simulink model "Aerodynamics4"  (R2017b)
settings: Solver=ode4  StartTime=0  StopTime=10.0  FixedStep=Ts  RelTol=1e-3
undefined symbols (not defined in the file or in its folder): Actuators, AeroDerivatives, Configuration, magnitude
libraries: aerolibatmos2 x1
settings Model: Creator=zht  LastModifiedBy=zht
settings DataIOCC: SaveFormat=StructureWithTime
settings OptimizationCC: BlockReduction=off  OptimizeBlockIOStorage=off  BufferReuse=off  GlobalBufferReuse=off  ExpressionFolding=off  LocalBlockOutputs=off
settings DebuggingCC: AlgebraicLoopMsg=none  UnconnectedInputMsg=none  UnconnectedOutputMsg=none  UnconnectedLineMsg=none

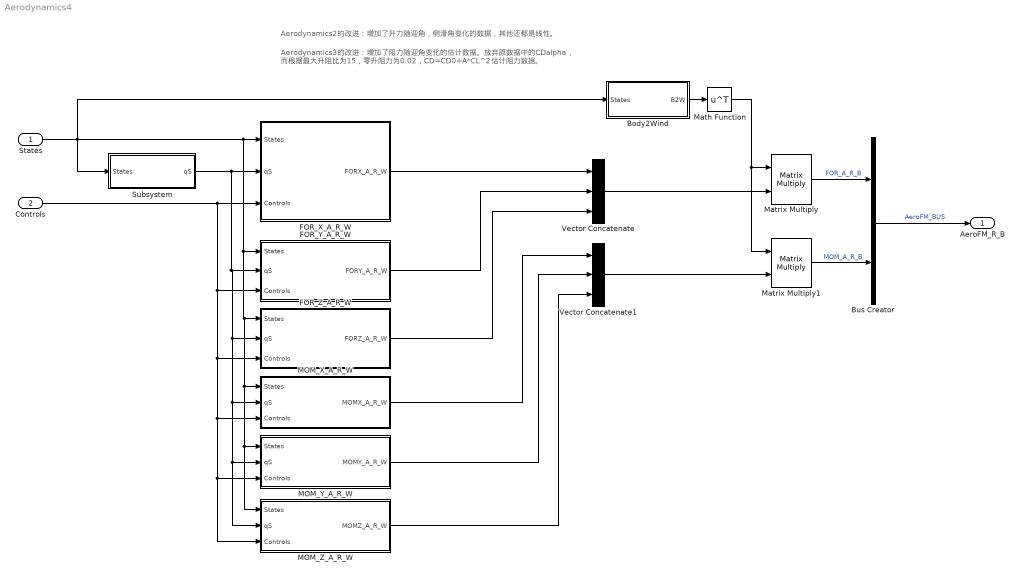
== system Aerodynamics4 ==
  note: Aerodynamics2的改进：增加了升力随迎角，侧滑角变化的数据，其他还都是线性。
  note: Aerodynamics3的改进：增加了阻力随迎角变化的估计数据。放弃原数据中的CDalpha，
      | 而根据最大升阻比为15，零升阻力为0.02，CD=CD0+A*CL^2估计阻力数据。
  States : Inport  OutDataTypeStr=Bus: States_BUS
  Controls : Inport  Port=2  OutDataTypeStr=Bus: Controls_CMD_BUS
  Body2Wind : Subsystem
  Bus Creator : BusCreator  Inputs=2  OutDataTypeStr=Bus: AeroFM_BUS
  FOR_X_A_R_W : Subsystem
  FOR_Y_A_R_W : Subsystem
  FOR_Z_A_R_W : Subsystem
  MOM_X_A_R_W : Subsystem
  MOM_Y_A_R_W : Subsystem
  MOM_Z_A_R_W : Subsystem
  Math Function : Math  Operator=transpose  SaturateOnIntegerOverflow=on
  Matrix Multiply : Product  Multiplication=Matrix(*)
  Matrix Multiply1 : Product  Multiplication=Matrix(*)
  Subsystem : Subsystem
  Vector Concatenate : Concatenate  NumInputs=3  Mode=Multidimensional array
  Vector Concatenate1 : Concatenate  NumInputs=3  Mode=Multidimensional array
  AeroFM_R_B : Outport  OutDataTypeStr=Bus: AeroFM_BUS
  wires:
  Bus Creator/1 -> AeroFM_R_B/1  "AeroFM_BUS"
  Controls/1 -> FOR_Y_A_R_W/3(Controls), FOR_Z_A_R_W/3(Controls), MOM_X_A_R_W/3(Controls), MOM_Y_A_R_W/3(Controls), MOM_Z_A_R_W/3(Controls), FOR_X_A_R_W/3(Controls)
  Vector Concatenate/1 -> Matrix Multiply/2
  Vector Concatenate1/1 -> Matrix Multiply1/2
  States/1 -> Subsystem/1(States), Body2Wind/1(States), MOM_Z_A_R_W/1(States), MOM_Y_A_R_W/1(States), MOM_X_A_R_W/1(States), FOR_Z_A_R_W/1(States), FOR_Y_A_R_W/1(States), FOR_X_A_R_W/1(States)
  Subsystem/1(qS) -> FOR_Z_A_R_W/2(qS), MOM_X_A_R_W/2(qS), MOM_Y_A_R_W/2(qS), MOM_Z_A_R_W/2(qS), FOR_Y_A_R_W/2(qS), FOR_X_A_R_W/2(qS)
  FOR_X_A_R_W/1(FORX_A_R_W) -> Vector Concatenate/1
  FOR_Y_A_R_W/1(FORY_A_R_W) -> Vector Concatenate/2
  FOR_Z_A_R_W/1(FORZ_A_R_W) -> Vector Concatenate/3
  MOM_X_A_R_W/1(MOMX_A_R_W) -> Vector Concatenate1/1
  MOM_Y_A_R_W/1(MOMY_A_R_W) -> Vector Concatenate1/2
  MOM_Z_A_R_W/1(MOMZ_A_R_W) -> Vector Concatenate1/3
  Body2Wind/1(B2W) -> Math Function/1
  Math Function/1 -> Matrix Multiply1/1, Matrix Multiply/1
  Matrix Multiply/1 -> Bus Creator/1  "FOR_A_R_B"
  Matrix Multiply1/1 -> Bus Creator/2  "MOM_A_R_B"

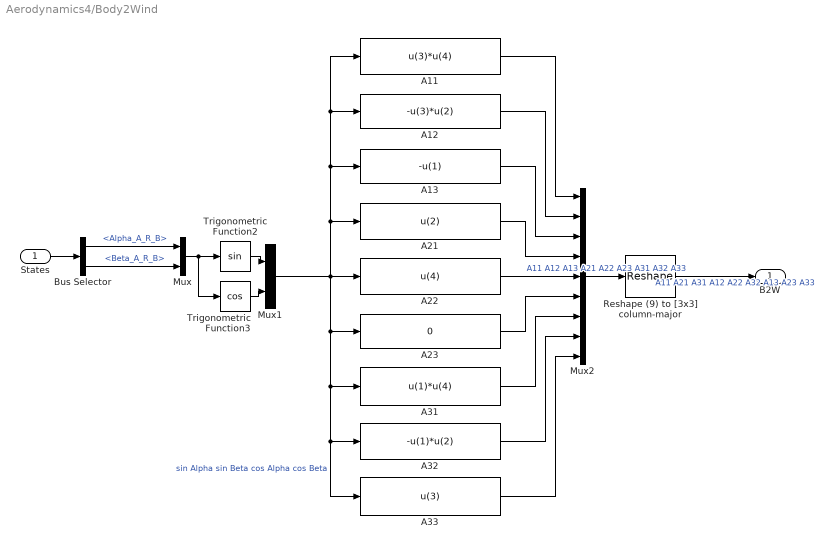
== system Aerodynamics4/Body2Wind ==
  States : Inport  OutDataTypeStr=Bus: States_BUS
  A11 : Fcn  Expr=u(3)*u(4)
  A12 : Fcn  Expr=-u(3)*u(2)
  A13 : Fcn  Expr=-u(1)
  A21 : Fcn  Expr=u(2)
  A22 : Fcn  Expr=u(4)
  A23 : Fcn  Expr=0
  A31 : Fcn  Expr=u(1)*u(4)
  A32 : Fcn  Expr=-u(1)*u(2)
  A33 : Fcn  Expr=u(3)
  Bus Selector : BusSelector  OutputSignals=Alpha_A_R_B,Beta_A_R_B
  Mux : Mux  Inputs=2
  Mux1 : Mux  Inputs=2
  Mux2 : Mux  Inputs=9
  Reshape (9) to [3x3] column-major : Reshape  OutputDimensionality=Customize  OutputDimensions=[3,3]
  Trigonometric Function2 : Trigonometry
  Trigonometric Function3 : Trigonometry  Operator=cos
  B2W : Outport  PortDimensions=[3 3]
  wires:
  Mux/1 -> Trigonometric Function2/1, Trigonometric Function3/1
  Trigonometric Function3/1 -> Mux1/2
  Trigonometric Function2/1 -> Mux1/1
  Bus Selector/2 -> Mux/2  "<Beta_A_R_B>"
  Bus Selector/1 -> Mux/1  "<Alpha_A_R_B>"
  States/1 -> Bus Selector/1
  A12/1 -> Mux2/2
  A13/1 -> Mux2/3
  A21/1 -> Mux2/4
  A32/1 -> Mux2/8
  A23/1 -> Mux2/6
  Mux2/1 -> Reshape (9) to [3x3] column-major/1  "A11 A12 A13 A21 A22 A23 A31 A32 A33"
  Reshape (9) to [3x3] column-major/1 -> B2W/1  "A11 A21 A31 A12 A22 A32 A13 A23 A33"
  A11/1 -> Mux2/1
  A22/1 -> Mux2/5
  A33/1 -> Mux2/9
  Mux1/1 -> A22/1, A23/1, A31/1, A32/1, A33/1, A21/1, A13/1, A11/1, A12/1  "sin Alpha sin Beta cos Alpha cos Beta"
  A31/1 -> Mux2/7

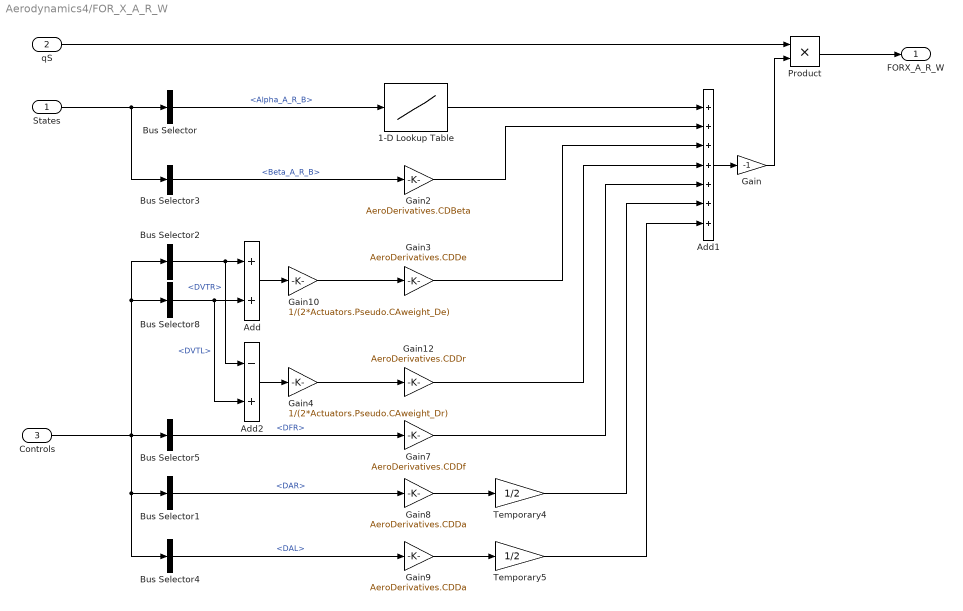
== system Aerodynamics4/FOR_X_A_R_W ==
  States : Inport  OutDataTypeStr=Bus: States_BUS  BusOutputAsStruct=on
  qS : Inport  Port=2  BusOutputAsStruct=on
  Controls : Inport  Port=3  OutDataTypeStr=Bus: Controls_CMD_BUS  BusOutputAsStruct=on
  1-D Lookup Table : Lookup_n-D  NumberOfTableDimensions=1  BreakpointsForDimension1=AeroDerivatives.CDa.alphaset  Table=AeroDerivatives.CDa.CDset  InternalRulePriority=Speed  RndMeth=Simplest  InputSameDT=on
  Add : Sum
  Add1 : Sum  Inputs=+++++++
  Add2 : Sum  Inputs=-+
  Bus Selector : BusSelector  OutputSignals=Alpha_A_R_B
  Bus Selector1 : BusSelector  OutputSignals=Actuators_CMD.DAR
  Bus Selector2 : BusSelector  OutputSignals=Actuators_CMD.DVTR
  Bus Selector3 : BusSelector  OutputSignals=Beta_A_R_B
  Bus Selector4 : BusSelector  OutputSignals=Actuators_CMD.DAL
  Bus Selector5 : BusSelector  OutputSignals=Actuators_CMD.DFR
  Bus Selector8 : BusSelector  OutputSignals=Actuators_CMD.DVTL
  Gain : Gain  Gain=-1
  Gain10 : Gain  Gain=1/(2*Actuators.Pseudo.CAweight_De)
  Gain12 : Gain  Gain=AeroDerivatives.CDDr
  Gain2 : Gain  Gain=AeroDerivatives.CDBeta
  Gain3 : Gain  Gain=AeroDerivatives.CDDe
  Gain4 : Gain  Gain=1/(2*Actuators.Pseudo.CAweight_Dr)
  Gain7 : Gain  Gain=AeroDerivatives.CDDf
  Gain8 : Gain  Gain=AeroDerivatives.CDDa
  Gain9 : Gain  Gain=AeroDerivatives.CDDa
  Product : Product
  Temporary4 : Gain  Gain=1/2
  Temporary5 : Gain  Gain=1/2
  FORX_A_R_W : Outport  Unit=N  PortDimensions=1
  wires:
  Bus Selector2/1 -> Add2/1, Add/1  "<DVTR>"
  Bus Selector8/1 -> Add2/2, Add/2  "<DVTL>"
  Gain2/1 -> Add1/2
  Product/1 -> FORX_A_R_W/1
  Controls/1 -> Bus Selector5/1, Bus Selector1/1, Bus Selector4/1, Bus Selector2/1, Bus Selector8/1
  1-D Lookup Table/1 -> Add1/1
  Gain3/1 -> Add1/3
  Gain/1 -> Product/2
  Gain4/1 -> Gain12/1
  States/1 -> Bus Selector3/1, Bus Selector/1
  Bus Selector5/1 -> Gain7/1  "<DFR>"
  Bus Selector/1 -> 1-D Lookup Table/1  "<Alpha_A_R_B>"
  Add1/1 -> Gain/1
  Bus Selector3/1 -> Gain2/1  "<Beta_A_R_B>"
  Bus Selector1/1 -> Gain8/1  "<DAR>"
  Bus Selector4/1 -> Gain9/1  "<DAL>"
  Gain8/1 -> Temporary4/1
  Gain9/1 -> Temporary5/1
  qS/1 -> Product/1
  Add/1 -> Gain10/1
  Gain10/1 -> Gain3/1
  Add2/1 -> Gain4/1
  Gain12/1 -> Add1/4
  Gain7/1 -> Add1/5
  Temporary4/1 -> Add1/6
  Temporary5/1 -> Add1/7

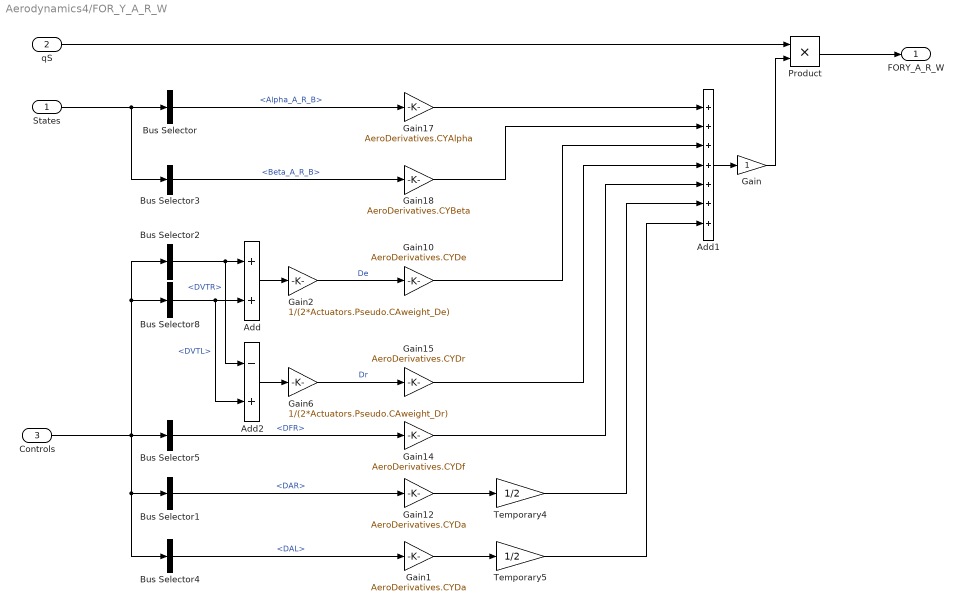
== system Aerodynamics4/FOR_Y_A_R_W ==
  States : Inport  OutDataTypeStr=Bus: States_BUS  BusOutputAsStruct=on
  qS : Inport  Port=2  BusOutputAsStruct=on
  Controls : Inport  Port=3  OutDataTypeStr=Bus: Controls_CMD_BUS  BusOutputAsStruct=on
  Add : Sum
  Add1 : Sum  Inputs=+++++++
  Add2 : Sum  Inputs=-+
  Bus Selector : BusSelector  OutputSignals=Alpha_A_R_B
  Bus Selector1 : BusSelector  OutputSignals=Actuators_CMD.DAR
  Bus Selector2 : BusSelector  OutputSignals=Actuators_CMD.DVTR
  Bus Selector3 : BusSelector  OutputSignals=Beta_A_R_B
  Bus Selector4 : BusSelector  OutputSignals=Actuators_CMD.DAL
  Bus Selector5 : BusSelector  OutputSignals=Actuators_CMD.DFR
  Bus Selector8 : BusSelector  OutputSignals=Actuators_CMD.DVTL
  Gain : Gain
  Gain1 : Gain  Gain=AeroDerivatives.CYDa
  Gain10 : Gain  Gain=AeroDerivatives.CYDe
  Gain12 : Gain  Gain=AeroDerivatives.CYDa
  Gain14 : Gain  Gain=AeroDerivatives.CYDf
  Gain15 : Gain  Gain=AeroDerivatives.CYDr
  Gain17 : Gain  Gain=AeroDerivatives.CYAlpha
  Gain18 : Gain  Gain=AeroDerivatives.CYBeta
  Gain2 : Gain  Gain=1/(2*Actuators.Pseudo.CAweight_De)
  Gain6 : Gain  Gain=1/(2*Actuators.Pseudo.CAweight_Dr)
  Product : Product
  Temporary4 : Gain  Gain=1/2
  Temporary5 : Gain  Gain=1/2
  FORY_A_R_W : Outport  Unit=N  PortDimensions=1
  wires:
  Bus Selector3/1 -> Gain18/1  "<Beta_A_R_B>"
  Gain12/1 -> Temporary4/1
  Gain18/1 -> Add1/2
  Gain2/1 -> Gain10/1  "De"
  qS/1 -> Product/1
  States/1 -> Bus Selector3/1, Bus Selector/1
  Add1/1 -> Gain/1
  Controls/1 -> Bus Selector5/1, Bus Selector1/1, Bus Selector4/1, Bus Selector2/1, Bus Selector8/1
  Bus Selector1/1 -> Gain12/1  "<DAR>"
  Gain1/1 -> Temporary5/1
  Gain/1 -> Product/2
  Bus Selector2/1 -> Add2/1, Add/1  "<DVTR>"
  Bus Selector/1 -> Gain17/1  "<Alpha_A_R_B>"
  Bus Selector5/1 -> Gain14/1  "<DFR>"
  Temporary5/1 -> Add1/7
  Temporary4/1 -> Add1/6
  Product/1 -> FORY_A_R_W/1
  Bus Selector4/1 -> Gain1/1  "<DAL>"
  Gain17/1 -> Add1/1
  Gain14/1 -> Add1/5
  Gain6/1 -> Gain15/1  "Dr"
  Gain15/1 -> Add1/4
  Add2/1 -> Gain6/1
  Bus Selector8/1 -> Add2/2, Add/2  "<DVTL>"
  Add/1 -> Gain2/1
  Gain10/1 -> Add1/3

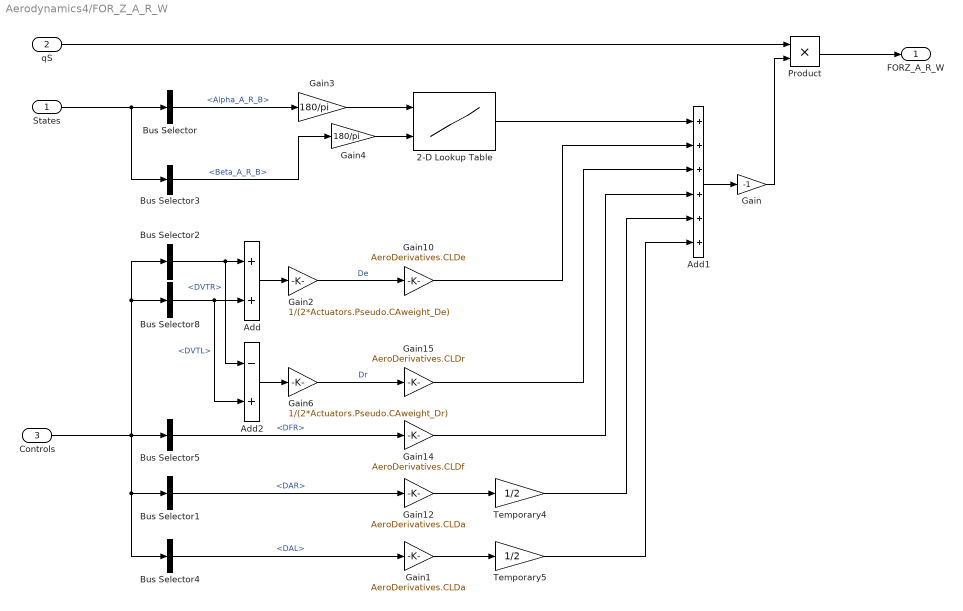
== system Aerodynamics4/FOR_Z_A_R_W ==
  States : Inport  OutDataTypeStr=Bus: States_BUS  BusOutputAsStruct=on
  qS : Inport  Port=2  BusOutputAsStruct=on
  Controls : Inport  Port=3  OutDataTypeStr=Bus: Controls_CMD_BUS  BusOutputAsStruct=on
  2-D Lookup Table : Lookup_n-D  BreakpointsForDimension1=AeroDerivatives.CLab.alphaset  BreakpointsForDimension2=AeroDerivatives.CLab.betaset  Table=AeroDerivatives.CLab.CLset'  InternalRulePriority=Speed  RndMeth=Simplest  InputSameDT=on
  Add : Sum
  Add1 : Sum  Inputs=++++++
  Add2 : Sum  Inputs=-+
  Bus Selector : BusSelector  OutputSignals=Alpha_A_R_B
  Bus Selector1 : BusSelector  OutputSignals=Actuators_CMD.DAR
  Bus Selector2 : BusSelector  OutputSignals=Actuators_CMD.DVTR
  Bus Selector3 : BusSelector  OutputSignals=Beta_A_R_B
  Bus Selector4 : BusSelector  OutputSignals=Actuators_CMD.DAL
  Bus Selector5 : BusSelector  OutputSignals=Actuators_CMD.DFR
  Bus Selector8 : BusSelector  OutputSignals=Actuators_CMD.DVTL
  Gain : Gain  Gain=-1
  Gain1 : Gain  Gain=AeroDerivatives.CLDa
  Gain10 : Gain  Gain=AeroDerivatives.CLDe
  Gain12 : Gain  Gain=AeroDerivatives.CLDa
  Gain14 : Gain  Gain=AeroDerivatives.CLDf
  Gain15 : Gain  Gain=AeroDerivatives.CLDr
  Gain2 : Gain  Gain=1/(2*Actuators.Pseudo.CAweight_De)
  Gain3 : Gain  Gain=180/pi
  Gain4 : Gain  Gain=180/pi
  Gain6 : Gain  Gain=1/(2*Actuators.Pseudo.CAweight_Dr)
  Product : Product
  Temporary4 : Gain  Gain=1/2
  Temporary5 : Gain  Gain=1/2
  FORZ_A_R_W : Outport  Unit=N  PortDimensions=1
  wires:
  Gain10/1 -> Add1/2
  Add/1 -> Gain2/1
  Bus Selector8/1 -> Add/2, Add2/2  "<DVTL>"
  Add2/1 -> Gain6/1
  Gain15/1 -> Add1/3
  Gain6/1 -> Gain15/1  "Dr"
  Gain14/1 -> Add1/4
  Bus Selector4/1 -> Gain1/1  "<DAL>"
  Product/1 -> FORZ_A_R_W/1
  Temporary4/1 -> Add1/5
  Temporary5/1 -> Add1/6
  Bus Selector5/1 -> Gain14/1  "<DFR>"
  Bus Selector/1 -> Gain3/1  "<Alpha_A_R_B>"
  Bus Selector2/1 -> Add/1, Add2/1  "<DVTR>"
  Gain/1 -> Product/2
  Gain1/1 -> Temporary5/1
  Bus Selector1/1 -> Gain12/1  "<DAR>"
  Controls/1 -> Bus Selector8/1, Bus Selector2/1, Bus Selector4/1, Bus Selector1/1, Bus Selector5/1
  Add1/1 -> Gain/1
  States/1 -> Bus Selector/1, Bus Selector3/1
  qS/1 -> Product/1
  Gain2/1 -> Gain10/1  "De"
  2-D Lookup Table/1 -> Add1/1
  Gain12/1 -> Temporary4/1
  Bus Selector3/1 -> Gain4/1  "<Beta_A_R_B>"
  Gain3/1 -> 2-D Lookup Table/1
  Gain4/1 -> 2-D Lookup Table/2

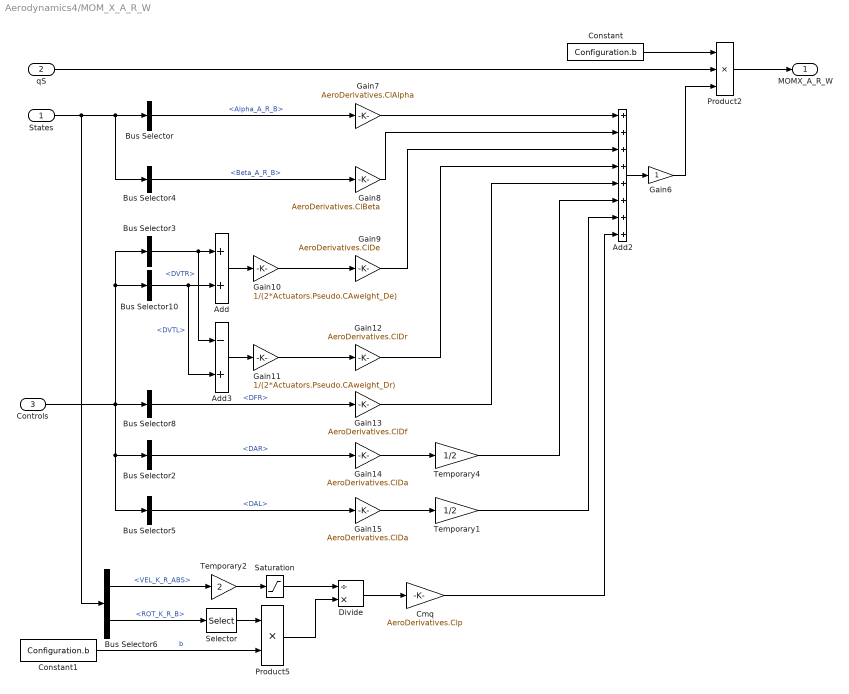
== system Aerodynamics4/MOM_X_A_R_W ==
  States : Inport  OutDataTypeStr=Bus: States_BUS  BusOutputAsStruct=on
  qS : Inport  Port=2  BusOutputAsStruct=on
  Controls : Inport  Port=3  OutDataTypeStr=Bus: Controls_CMD_BUS  BusOutputAsStruct=on
  Add : Sum
  Add2 : Sum  Inputs=++++++++
  Add3 : Sum  Inputs=-+
  Bus Selector : BusSelector  OutputSignals=Alpha_A_R_B
  Bus Selector10 : BusSelector  OutputSignals=Actuators_CMD.DVTL
  Bus Selector2 : BusSelector  OutputSignals=Actuators_CMD.DAR
  Bus Selector3 : BusSelector  OutputSignals=Actuators_CMD.DVTR
  Bus Selector4 : BusSelector  OutputSignals=Beta_A_R_B
  Bus Selector5 : BusSelector  OutputSignals=Actuators_CMD.DAL
  Bus Selector6 : BusSelector  OutputSignals=VEL_K_R_ABS,ROT_K_R_B
  Bus Selector8 : BusSelector  OutputSignals=Actuators_CMD.DFR
  Cmq : Gain  Gain=AeroDerivatives.Clp
  Constant : Constant  Value=Configuration.b
  Constant1 : Constant  Value=Configuration.b
  Divide : Product  Inputs=/*
  Gain10 : Gain  Gain=1/(2*Actuators.Pseudo.CAweight_De)
  Gain11 : Gain  Gain=1/(2*Actuators.Pseudo.CAweight_Dr)
  Gain12 : Gain  Gain=AeroDerivatives.ClDr
  Gain13 : Gain  Gain=AeroDerivatives.ClDf
  Gain14 : Gain  Gain=AeroDerivatives.ClDa
  Gain15 : Gain  Gain=AeroDerivatives.ClDa
  Gain6 : Gain
  Gain7 : Gain  Gain=AeroDerivatives.ClAlpha
  Gain8 : Gain  Gain=AeroDerivatives.ClBeta
  Gain9 : Gain  Gain=AeroDerivatives.ClDe
  Product2 : Product  Inputs=3
  Product5 : Product
  Saturation : Saturate  UpperLimit=inf  LowerLimit=10
  Selector : Selector  InputPortWidth=3  IndexOptions=Index vector (dialog)  Indices=[1]  OutputSizes=1
  Temporary1 : Gain  Gain=1/2
  Temporary2 : Gain  Gain=2
  Temporary4 : Gain  Gain=1/2
  MOMX_A_R_W : Outport  Unit=N  PortDimensions=1
  wires:
  Bus Selector4/1 -> Gain8/1  "<Beta_A_R_B>"
  Gain14/1 -> Temporary4/1
  Gain8/1 -> Add2/2
  Gain10/1 -> Gain9/1
  qS/1 -> Product2/2
  States/1 -> Bus Selector6/1, Bus Selector4/1, Bus Selector/1
  Add2/1 -> Gain6/1
  Controls/1 -> Bus Selector8/1, Bus Selector2/1, Bus Selector5/1, Bus Selector3/1, Bus Selector10/1
  Bus Selector2/1 -> Gain14/1  "<DAR>"
  Gain15/1 -> Temporary1/1
  Gain6/1 -> Product2/3
  Bus Selector3/1 -> Add3/1, Add/1  "<DVTR>"
  Bus Selector/1 -> Gain7/1  "<Alpha_A_R_B>"
  Bus Selector8/1 -> Gain13/1  "<DFR>"
  Temporary1/1 -> Add2/7
  Temporary4/1 -> Add2/6
  Product2/1 -> MOMX_A_R_W/1
  Bus Selector5/1 -> Gain15/1  "<DAL>"
  Gain7/1 -> Add2/1
  Gain13/1 -> Add2/5
  Gain11/1 -> Gain12/1
  Gain12/1 -> Add2/4
  Add3/1 -> Gain11/1
  Bus Selector10/1 -> Add3/2, Add/2  "<DVTL>"
  Add/1 -> Gain10/1
  Gain9/1 -> Add2/3
  Constant/1 -> Product2/1
  Product5/1 -> Divide/2
  Saturation/1 -> Divide/1
  Constant1/1 -> Product5/2  "b"
  Selector/1 -> Product5/1
  Temporary2/1 -> Saturation/1
  Divide/1 -> Cmq/1
  Bus Selector6/1 -> Temporary2/1  "<VEL_K_R_ABS>"
  Bus Selector6/2 -> Selector/1  "<ROT_K_R_B>"
  Cmq/1 -> Add2/8

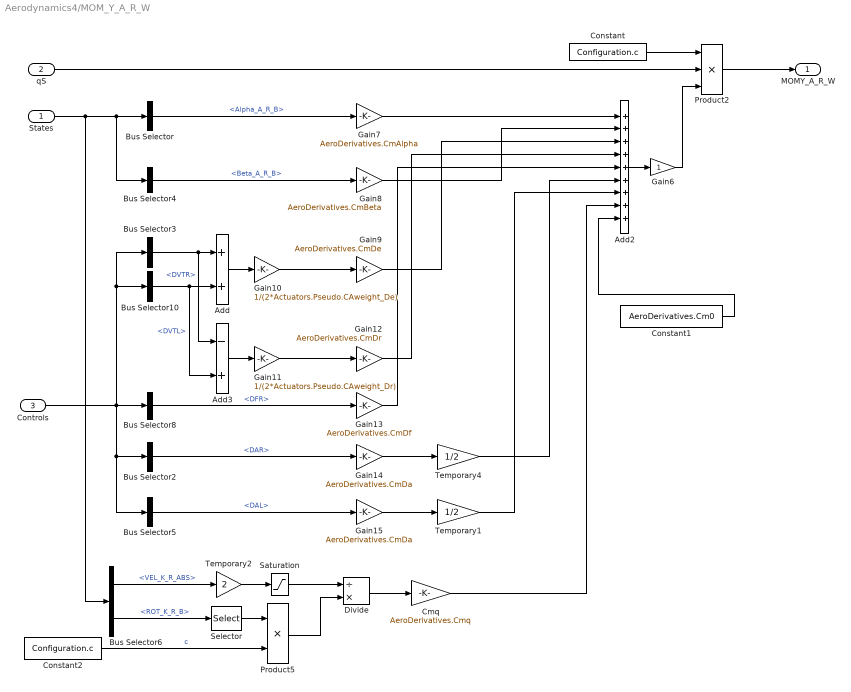
== system Aerodynamics4/MOM_Y_A_R_W ==
  States : Inport  OutDataTypeStr=Bus: States_BUS  BusOutputAsStruct=on
  qS : Inport  Port=2  BusOutputAsStruct=on
  Controls : Inport  Port=3  OutDataTypeStr=Bus: Controls_CMD_BUS  BusOutputAsStruct=on
  Add : Sum
  Add2 : Sum  Inputs=+++++++++
  Add3 : Sum  Inputs=-+
  Bus Selector : BusSelector  OutputSignals=Alpha_A_R_B
  Bus Selector10 : BusSelector  OutputSignals=Actuators_CMD.DVTL
  Bus Selector2 : BusSelector  OutputSignals=Actuators_CMD.DAR
  Bus Selector3 : BusSelector  OutputSignals=Actuators_CMD.DVTR
  Bus Selector4 : BusSelector  OutputSignals=Beta_A_R_B
  Bus Selector5 : BusSelector  OutputSignals=Actuators_CMD.DAL
  Bus Selector6 : BusSelector  OutputSignals=VEL_K_R_ABS,ROT_K_R_B
  Bus Selector8 : BusSelector  OutputSignals=Actuators_CMD.DFR
  Cmq : Gain  Gain=AeroDerivatives.Cmq
  Constant : Constant  Value=Configuration.c
  Constant1 : Constant  Value=AeroDerivatives.Cm0
  Constant2 : Constant  Value=Configuration.c
  Divide : Product  Inputs=/*
  Gain10 : Gain  Gain=1/(2*Actuators.Pseudo.CAweight_De)
  Gain11 : Gain  Gain=1/(2*Actuators.Pseudo.CAweight_Dr)
  Gain12 : Gain  Gain=AeroDerivatives.CmDr
  Gain13 : Gain  Gain=AeroDerivatives.CmDf
  Gain14 : Gain  Gain=AeroDerivatives.CmDa
  Gain15 : Gain  Gain=AeroDerivatives.CmDa
  Gain6 : Gain
  Gain7 : Gain  Gain=AeroDerivatives.CmAlpha
  Gain8 : Gain  Gain=AeroDerivatives.CmBeta
  Gain9 : Gain  Gain=AeroDerivatives.CmDe
  Product2 : Product  Inputs=3
  Product5 : Product
  Saturation : Saturate  UpperLimit=inf  LowerLimit=10
  Selector : Selector  InputPortWidth=3  IndexOptions=Index vector (dialog)  Indices=[2]  OutputSizes=1
  Temporary1 : Gain  Gain=1/2
  Temporary2 : Gain  Gain=2
  Temporary4 : Gain  Gain=1/2
  MOMY_A_R_W : Outport  Unit=N  PortDimensions=1
  wires:
  Gain9/1 -> Add2/3
  Add/1 -> Gain10/1
  Bus Selector10/1 -> Add/2, Add3/2  "<DVTL>"
  Add3/1 -> Gain11/1
  Gain12/1 -> Add2/4
  Gain11/1 -> Gain12/1
  Gain13/1 -> Add2/5
  Gain7/1 -> Add2/1
  Bus Selector5/1 -> Gain15/1  "<DAL>"
  Product2/1 -> MOMY_A_R_W/1
  Temporary4/1 -> Add2/6
  Temporary1/1 -> Add2/7
  Bus Selector8/1 -> Gain13/1  "<DFR>"
  Bus Selector/1 -> Gain7/1  "<Alpha_A_R_B>"
  Bus Selector3/1 -> Add/1, Add3/1  "<DVTR>"
  Gain6/1 -> Product2/3
  Gain15/1 -> Temporary1/1
  Bus Selector2/1 -> Gain14/1  "<DAR>"
  Controls/1 -> Bus Selector10/1, Bus Selector3/1, Bus Selector5/1, Bus Selector2/1, Bus Selector8/1
  Add2/1 -> Gain6/1
  qS/1 -> Product2/2
  Gain10/1 -> Gain9/1
  Gain8/1 -> Add2/2
  Gain14/1 -> Temporary4/1
  Bus Selector4/1 -> Gain8/1  "<Beta_A_R_B>"
  Constant/1 -> Product2/1
  Constant1/1 -> Add2/9
  Temporary2/1 -> Saturation/1
  Selector/1 -> Product5/1
  Product5/1 -> Divide/2
  Bus Selector6/2 -> Selector/1  "<ROT_K_R_B>"
  Cmq/1 -> Add2/8
  Divide/1 -> Cmq/1
  Saturation/1 -> Divide/1
  Bus Selector6/1 -> Temporary2/1  "<VEL_K_R_ABS>"
  States/1 -> Bus Selector6/1, Bus Selector/1, Bus Selector4/1
  Constant2/1 -> Product5/2  "c"

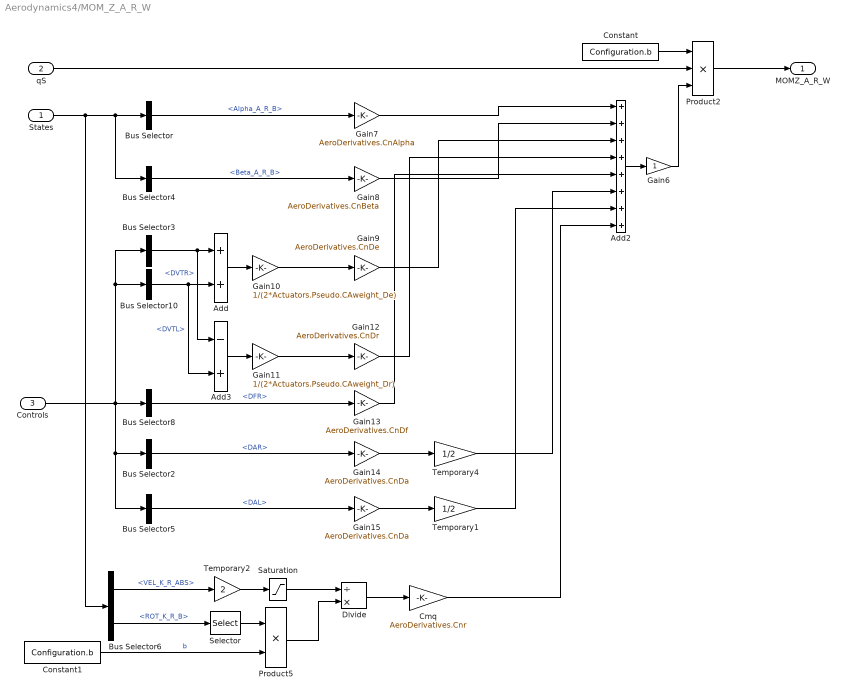
== system Aerodynamics4/MOM_Z_A_R_W ==
  States : Inport  OutDataTypeStr=Bus: States_BUS  BusOutputAsStruct=on
  qS : Inport  Port=2  BusOutputAsStruct=on
  Controls : Inport  Port=3  OutDataTypeStr=Bus: Controls_CMD_BUS  BusOutputAsStruct=on
  Add : Sum
  Add2 : Sum  Inputs=++++++++
  Add3 : Sum  Inputs=-+
  Bus Selector : BusSelector  OutputSignals=Alpha_A_R_B
  Bus Selector10 : BusSelector  OutputSignals=Actuators_CMD.DVTL
  Bus Selector2 : BusSelector  OutputSignals=Actuators_CMD.DAR
  Bus Selector3 : BusSelector  OutputSignals=Actuators_CMD.DVTR
  Bus Selector4 : BusSelector  OutputSignals=Beta_A_R_B
  Bus Selector5 : BusSelector  OutputSignals=Actuators_CMD.DAL
  Bus Selector6 : BusSelector  OutputSignals=VEL_K_R_ABS,ROT_K_R_B
  Bus Selector8 : BusSelector  OutputSignals=Actuators_CMD.DFR
  Cmq : Gain  Gain=AeroDerivatives.Cnr
  Constant : Constant  Value=Configuration.b
  Constant1 : Constant  Value=Configuration.b
  Divide : Product  Inputs=/*
  Gain10 : Gain  Gain=1/(2*Actuators.Pseudo.CAweight_De)
  Gain11 : Gain  Gain=1/(2*Actuators.Pseudo.CAweight_Dr)
  Gain12 : Gain  Gain=AeroDerivatives.CnDr
  Gain13 : Gain  Gain=AeroDerivatives.CnDf
  Gain14 : Gain  Gain=AeroDerivatives.CnDa
  Gain15 : Gain  Gain=AeroDerivatives.CnDa
  Gain6 : Gain
  Gain7 : Gain  Gain=AeroDerivatives.CnAlpha
  Gain8 : Gain  Gain=AeroDerivatives.CnBeta
  Gain9 : Gain  Gain=AeroDerivatives.CnDe
  Product2 : Product  Inputs=3
  Product5 : Product
  Saturation : Saturate  UpperLimit=inf  LowerLimit=10
  Selector : Selector  InputPortWidth=3  IndexOptions=Index vector (dialog)  Indices=[3]  OutputSizes=1
  Temporary1 : Gain  Gain=1/2
  Temporary2 : Gain  Gain=2
  Temporary4 : Gain  Gain=1/2
  MOMZ_A_R_W : Outport  Unit=N  PortDimensions=1
  wires:
  Bus Selector4/1 -> Gain8/1  "<Beta_A_R_B>"
  Gain14/1 -> Temporary4/1
  Gain8/1 -> Add2/2
  Gain10/1 -> Gain9/1
  qS/1 -> Product2/2
  Add2/1 -> Gain6/1
  Controls/1 -> Bus Selector8/1, Bus Selector2/1, Bus Selector5/1, Bus Selector3/1, Bus Selector10/1
  Bus Selector2/1 -> Gain14/1  "<DAR>"
  Gain15/1 -> Temporary1/1
  Gain6/1 -> Product2/3
  Bus Selector3/1 -> Add3/1, Add/1  "<DVTR>"
  Bus Selector/1 -> Gain7/1  "<Alpha_A_R_B>"
  Bus Selector8/1 -> Gain13/1  "<DFR>"
  Temporary1/1 -> Add2/7
  Temporary4/1 -> Add2/6
  Product2/1 -> MOMZ_A_R_W/1
  Bus Selector5/1 -> Gain15/1  "<DAL>"
  Gain7/1 -> Add2/1
  Gain13/1 -> Add2/5
  Gain11/1 -> Gain12/1
  Gain12/1 -> Add2/4
  Add3/1 -> Gain11/1
  Bus Selector10/1 -> Add3/2, Add/2  "<DVTL>"
  Add/1 -> Gain10/1
  Gain9/1 -> Add2/3
  Constant/1 -> Product2/1
  Temporary2/1 -> Saturation/1
  Selector/1 -> Product5/1
  Product5/1 -> Divide/2
  Bus Selector6/2 -> Selector/1  "<ROT_K_R_B>"
  Cmq/1 -> Add2/8
  Divide/1 -> Cmq/1
  Saturation/1 -> Divide/1
  Bus Selector6/1 -> Temporary2/1  "<VEL_K_R_ABS>"
  States/1 -> Bus Selector6/1, Bus Selector4/1, Bus Selector/1
  Constant1/1 -> Product5/2  "b"

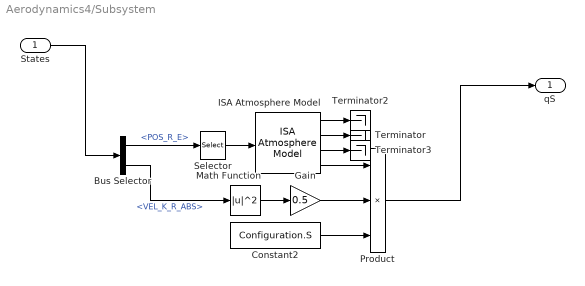
== system Aerodynamics4/Subsystem ==
  States : Inport
  Bus Selector : BusSelector  OutputSignals=POS_R_E,VEL_K_R_ABS
  Constant2 : Constant  Value=Configuration.S
  Gain : Gain  Gain=0.5
  ISA Atmosphere Model : aerolibatmos2/ISA Atmosphere Model  custom=off  g=9.80665  gamma=1.4  R=287.0531  L=0.0065  h_trop=11000  h_strat=20000  rho0=1.225  P0=101325  T0=288.15  h0=0
      settings: SourceProductName=Aerospace Blockset
  Math Function : Math  Operator=magnitude^2  SaturateOnIntegerOverflow=on
  Product : Product  Inputs=3
  Selector : Selector  InputPortWidth=3  IndexOptions=Index vector (dialog)  Indices=[3]  OutputSizes=1
  Terminator : Terminator
  Terminator2 : Terminator
  Terminator3 : Terminator
  qS : Outport
  wires:
  Selector/1 -> ISA Atmosphere Model/1
  ISA Atmosphere Model/1 -> Terminator2/1
  ISA Atmosphere Model/3 -> Terminator3/1
  States/1 -> Bus Selector/1
  Bus Selector/1 -> Selector/1  "<POS_R_E>"
  ISA Atmosphere Model/2 -> Terminator/1
  Constant2/1 -> Product/3
  ISA Atmosphere Model/4 -> Product/1
  Gain/1 -> Product/2
  Product/1 -> qS/1
  Math Function/1 -> Gain/1
  Bus Selector/2 -> Math Function/1  "<VEL_K_R_ABS>"
